simulink model "Laengsdynamik_V1"  (R2016a)
settings: Solver=ode1  StartTime=0.0  StopTime=70  FixedStep=0.01  RelTol=1e-3
undefined symbols (not defined in the file): A, cW, fr0, fr1, fr4, g, i, iHA, m, Mmot, nMot, rho, rRad, v12, v23, v34, v45, Winkel_DK
libraries: simulink x1
settings Model: Creator=Michaél  LastModifiedBy=Michaél

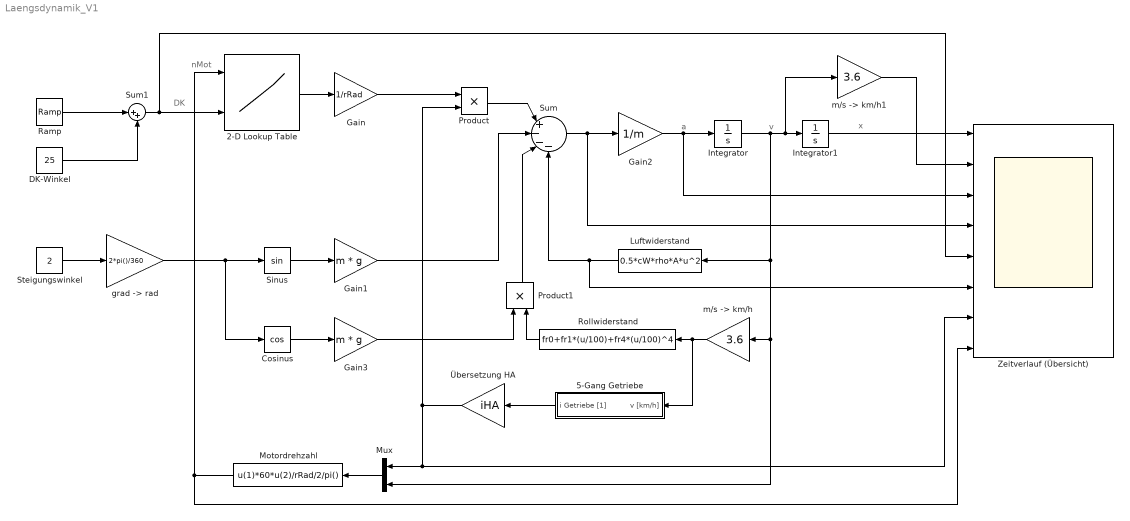
== system Laengsdynamik_V1 ==
  note: a
  note: x
  note: v
  note: DK
  note: nMot
  2-D Lookup Table : Lookup_n-D  BreakpointsForDimension1=nMot  BreakpointsForDimension2=Winkel_DK  Table=Mmot  InternalRulePriority=Speed  RndMeth=Simplest  InputSameDT=on
  5-Gang Getriebe : Subsystem
  Cosinus : Trigonometry  Operator=cos
  DK-Winkel : Constant  Value=25
  Gain : Gain  Gain=1/rRad
  Gain1 : Gain  Gain=m * g
  Gain2 : Gain  Gain=1/m
  Gain3 : Gain  Gain=m * g
  Integrator : Integrator
  Integrator1 : Integrator
  Luftwiderstand : Fcn  Expr=0.5*cW*rho*A*u^2
  Motordrehzahl : Fcn  Expr=u(1)*60*u(2)/rRad/2/pi()
  Mux : Mux  Inputs=2
  Product : Product
  Product1 : Product
  Ramp : simulink/Sources/Ramp  slope=0.5  start=0  X0=0
  Rollwiderstand : Fcn  Expr=fr0+fr1*(u/100)+fr4*(u/100)^4
  Sinus : Trigonometry
  Steigungswinkel : Constant  Value=2
  Sum : Sum  Inputs=|+---
  Sum1 : Sum  Inputs=|++
  Zeitverlauf (Übersicht) : Scope  NumInputPorts=8
  "grad -> rad" : Gain  Gain=2*pi()/360
  "m/s -> km/h" : Gain  Gain=3.6
  "m/s -> km/h1" : Gain  Gain=3.6
  Übersetzung HA : Gain  Gain=iHA
  wires:
  2-D Lookup Table/1 -> Gain/1
  Gain/1 -> Product/1
  Product/1 -> Sum/1
  Steigungswinkel/1 -> "grad -> rad"/1
  Sum/1 -> Zeitverlauf (Übersicht)/4, Gain2/1
  Gain2/1 -> Zeitverlauf (Übersicht)/3, Integrator/1
  Luftwiderstand/1 -> Zeitverlauf (Übersicht)/6, Sum/4
  Sinus/1 -> Gain1/1
  Rollwiderstand/1 -> Product1/2
  "m/s -> km/h"/1 -> 5-Gang Getriebe/1(v [km/h]), Rollwiderstand/1
  Cosinus/1 -> Gain3/1
  Product1/1 -> Sum/3
  Integrator1/1 -> Zeitverlauf (Übersicht)/1
  5-Gang Getriebe/1(i Getriebe [1]) -> Übersetzung HA/1
  Übersetzung HA/1 -> Zeitverlauf (Übersicht)/7, Mux/1, Product/2
  Mux/1 -> Motordrehzahl/1
  Sum1/1 -> Zeitverlauf (Übersicht)/5, 2-D Lookup Table/2
  Ramp/1 -> Sum1/1
  DK-Winkel/1 -> Sum1/2
  Integrator/1 -> Mux/2, "m/s -> km/h"/1, Luftwiderstand/1, "m/s -> km/h1"/1, Integrator1/1
  "m/s -> km/h1"/1 -> Zeitverlauf (Übersicht)/2
  Gain1/1 -> Sum/2
  Gain3/1 -> Product1/1
  "grad -> rad"/1 -> Sinus/1, Cosinus/1
  Motordrehzahl/1 -> 2-D Lookup Table/1, Zeitverlauf (Übersicht)/8

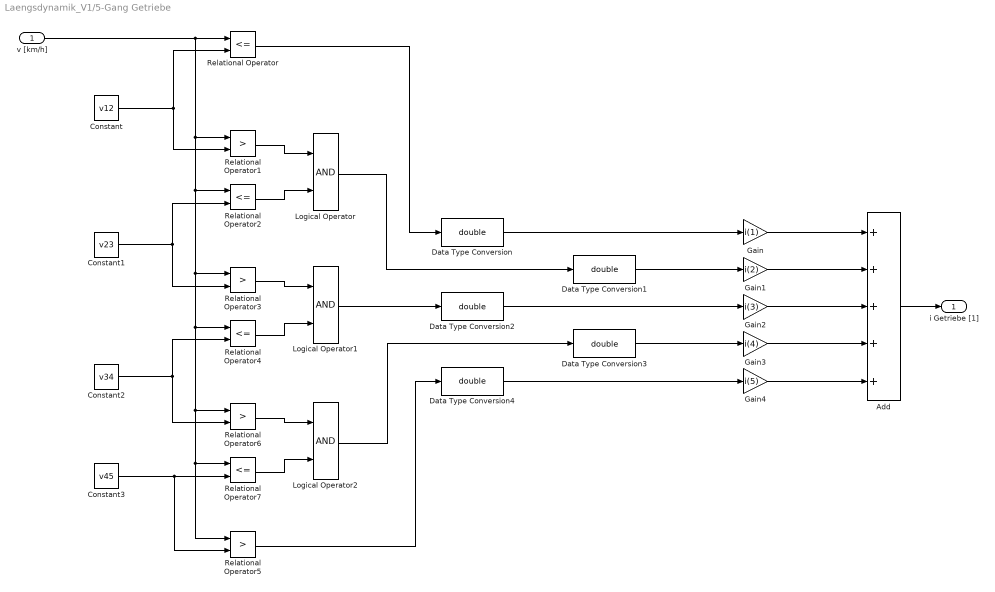
== system Laengsdynamik_V1/5-Gang Getriebe ==
  v [km/h] : Inport
  Add : Sum  Inputs=+++++
  Constant : Constant  Value=v12
  Constant1 : Constant  Value=v23
  Constant2 : Constant  Value=v34
  Constant3 : Constant  Value=v45
  Data Type Conversion{,1..4} (5 alike) : DataTypeConversion  OutDataTypeStr=double
  Gain : Gain  Gain=i(1)
  Gain1 : Gain  Gain=i(2)
  Gain2 : Gain  Gain=i(3)
  Gain3 : Gain  Gain=i(4)
  Gain4 : Gain  Gain=i(5)
  Logical Operator : Logic  AllPortsSameDT=off  OutDataTypeStr=boolean
  Logical Operator1 : Logic  AllPortsSameDT=off  OutDataTypeStr=boolean
  Logical Operator2 : Logic  AllPortsSameDT=off  OutDataTypeStr=boolean
  Relational Operator{,2,4,7} (4 alike) : RelationalOperator  Operator=<=  OutDataTypeStr=boolean
  Relational Operator{1,3,5..6} (4 alike) : RelationalOperator  Operator=>  OutDataTypeStr=boolean
  i Getriebe [1] : Outport
  wires:
  Constant/1 -> Relational Operator1/2, Relational Operator/2
  v [km/h]/1 -> Relational Operator3/1, Relational Operator6/1, Relational Operator7/1, Relational Operator5/1, Relational Operator4/1, Relational Operator2/1, Relational Operator1/1, Relational Operator/1
  Constant1/1 -> Relational Operator2/2, Relational Operator3/2
  Constant2/1 -> Relational Operator4/2, Relational Operator6/2
  Constant3/1 -> Relational Operator7/2, Relational Operator5/2
  Relational Operator1/1 -> Logical Operator/1
  Relational Operator2/1 -> Logical Operator/2
  Relational Operator3/1 -> Logical Operator1/1
  Relational Operator4/1 -> Logical Operator1/2
  Relational Operator6/1 -> Logical Operator2/1
  Relational Operator7/1 -> Logical Operator2/2
  Logical Operator1/1 -> Data Type Conversion2/1
  Logical Operator/1 -> Data Type Conversion1/1
  Relational Operator/1 -> Data Type Conversion/1
  Logical Operator2/1 -> Data Type Conversion3/1
  Relational Operator5/1 -> Data Type Conversion4/1
  Add/1 -> i Getriebe [1]/1
  Data Type Conversion/1 -> Gain/1
  Data Type Conversion1/1 -> Gain1/1
  Data Type Conversion2/1 -> Gain2/1
  Data Type Conversion3/1 -> Gain3/1
  Data Type Conversion4/1 -> Gain4/1
  Gain1/1 -> Add/2
  Gain/1 -> Add/1
  Gain2/1 -> Add/3
  Gain3/1 -> Add/4
  Gain4/1 -> Add/5
